simulink model "Hand"  (R2023b)
settings: Solver=ode45  StartTime=0.0  StopTime=100  RelTol=1e-3  EnableMultiTasking=on
model workspace (MAT data in the model file):
  InitialAngle = 0
libraries: simulink x22, vrlib x16, sharedtransform x15
(part 2 of 2)

== system Hand/Subsystem3/Angle To Orientation1 ==
  Y : Inport
  X : Inport  Port=2
  Z : Inport  Port=3
  Multiplier3 : Constant  Value=-1
  Product : Product
  Rotation Angles : Concatenate  NumInputs=3  Mode=Multidimensional array
  Rotation Angles to Direction Cosine Matrix : sharedtransform/Rotation Angles to Direction Cosine Matrix  rotationOrder=XYZ  aMode=aMode
  Rotation Matrix to VR Rotation : vrlib/Utilities/Rotation Matrix to VR Rotation  maxzero=1e-12
  Out1 : Outport
  wires:
  Product/1 -> Rotation Angles to Direction Cosine Matrix/1
  Multiplier3/1 -> Product/1
  Y/1 -> Rotation Angles/2
  Rotation Angles to Direction Cosine Matrix/1 -> Rotation Matrix to VR Rotation/1
  Rotation Matrix to VR Rotation/1 -> Out1/1
  Rotation Angles/1 -> Product/2
  X/1 -> Rotation Angles/1
  Z/1 -> Rotation Angles/3

== system Hand/Subsystem3/Angle To Orientation2 ==
  Y : Inport
  X : Inport  Port=2
  Z : Inport  Port=3
  Multiplier3 : Constant  Value=-1
  Product : Product
  Rotation Angles : Concatenate  NumInputs=3  Mode=Multidimensional array
  Rotation Angles to Direction Cosine Matrix : sharedtransform/Rotation Angles to Direction Cosine Matrix  rotationOrder=XYZ  aMode=aMode
  Rotation Matrix to VR Rotation : vrlib/Utilities/Rotation Matrix to VR Rotation  maxzero=1e-12
  Out1 : Outport
  wires:
  Product/1 -> Rotation Angles to Direction Cosine Matrix/1
  Multiplier3/1 -> Product/1
  Y/1 -> Rotation Angles/2
  Rotation Angles to Direction Cosine Matrix/1 -> Rotation Matrix to VR Rotation/1
  Rotation Matrix to VR Rotation/1 -> Out1/1
  Rotation Angles/1 -> Product/2
  X/1 -> Rotation Angles/1
  Z/1 -> Rotation Angles/3

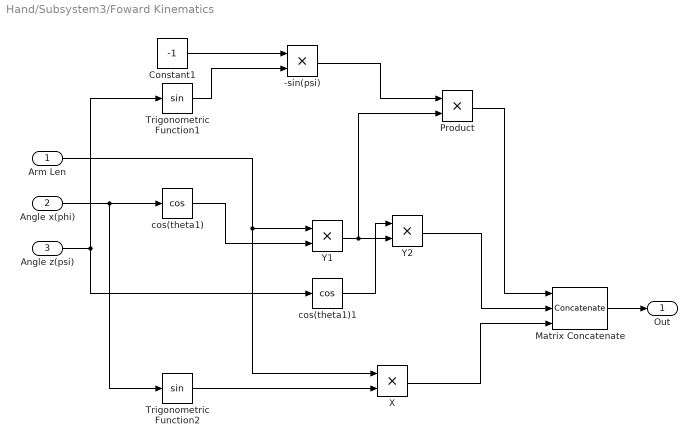
== system Hand/Subsystem3/Foward Kinematics ==
  Arm Len : Inport
  Angle x(phi) : Inport  Port=2
  Angle z(psi) : Inport  Port=3
  -sin(psi) : Product
  Constant1 : Constant  Value=-1
  Matrix Concatenate : Concatenate  NumInputs=3  ConcatenateDimension=2
  Product : Product
  Trigonometric Function1 : Trigonometry  OutputSignalType=real
  Trigonometric Function2 : Trigonometry  OutputSignalType=real
  X : Product
  Y1 : Product
  Y2 : Product
  cos(theta1) : Trigonometry  Operator=cos
  cos(theta1)1 : Trigonometry  Operator=cos
  Out : Outport
  wires:
  Matrix Concatenate/1 -> Out/1
  X/1 -> Matrix Concatenate/3
  Arm Len/1 -> X/1, Y1/1
  Trigonometric Function2/1 -> X/2
  Y1/1 -> Product/2, Y2/2
  cos(theta1)1/1 -> Y2/1
  Y2/1 -> Matrix Concatenate/2
  Product/1 -> Matrix Concatenate/1
  Constant1/1 -> -sin(psi)/1
  Trigonometric Function1/1 -> -sin(psi)/2
  Angle x(phi)/1 -> Trigonometric Function2/1, cos(theta1)/1
  cos(theta1)/1 -> Y1/2
  Angle z(psi)/1 -> Trigonometric Function1/1, cos(theta1)1/1
  -sin(psi)/1 -> Product/1

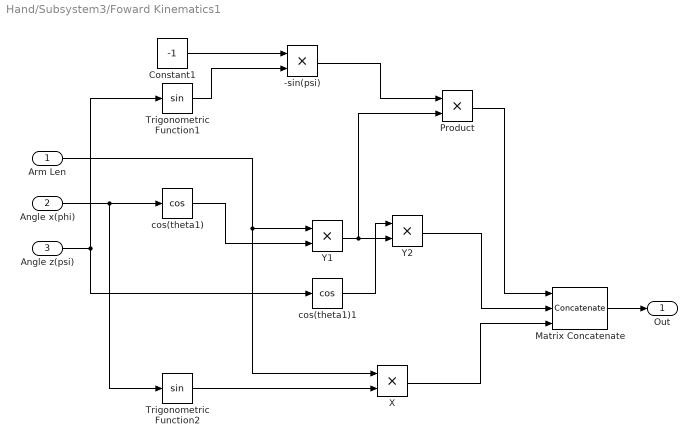
== system Hand/Subsystem3/Foward Kinematics1 ==
  Arm Len : Inport
  Angle x(phi) : Inport  Port=2
  Angle z(psi) : Inport  Port=3
  -sin(psi) : Product
  Constant1 : Constant  Value=-1
  Matrix Concatenate : Concatenate  NumInputs=3  ConcatenateDimension=2
  Product : Product
  Trigonometric Function1 : Trigonometry  OutputSignalType=real
  Trigonometric Function2 : Trigonometry  OutputSignalType=real
  X : Product
  Y1 : Product
  Y2 : Product
  cos(theta1) : Trigonometry  Operator=cos
  cos(theta1)1 : Trigonometry  Operator=cos
  Out : Outport
  wires:
  Matrix Concatenate/1 -> Out/1
  X/1 -> Matrix Concatenate/3
  Arm Len/1 -> X/1, Y1/1
  Trigonometric Function2/1 -> X/2
  Y1/1 -> Product/2, Y2/2
  cos(theta1)1/1 -> Y2/1
  Y2/1 -> Matrix Concatenate/2
  Product/1 -> Matrix Concatenate/1
  Constant1/1 -> -sin(psi)/1
  Trigonometric Function1/1 -> -sin(psi)/2
  Angle x(phi)/1 -> Trigonometric Function2/1, cos(theta1)/1
  cos(theta1)/1 -> Y1/2
  Angle z(psi)/1 -> Trigonometric Function1/1, cos(theta1)1/1
  -sin(psi)/1 -> Product/1

== system Hand/Subsystem4/Angle To Orientation ==
  Y : Inport
  X : Inport  Port=2
  Z : Inport  Port=3
  Multiplier3 : Constant  Value=-1
  Product : Product
  Rotation Angles : Concatenate  NumInputs=3  Mode=Multidimensional array
  Rotation Angles to Direction Cosine Matrix : sharedtransform/Rotation Angles to Direction Cosine Matrix  rotationOrder=XYZ  aMode=aMode
  Rotation Matrix to VR Rotation : vrlib/Utilities/Rotation Matrix to VR Rotation  maxzero=1e-12
  Out1 : Outport
  wires:
  Product/1 -> Rotation Angles to Direction Cosine Matrix/1
  Multiplier3/1 -> Product/1
  Y/1 -> Rotation Angles/2
  Rotation Angles to Direction Cosine Matrix/1 -> Rotation Matrix to VR Rotation/1
  Rotation Matrix to VR Rotation/1 -> Out1/1
  Rotation Angles/1 -> Product/2
  X/1 -> Rotation Angles/1
  Z/1 -> Rotation Angles/3

== system Hand/Subsystem4/Angle To Orientation1 ==
  Y : Inport
  X : Inport  Port=2
  Z : Inport  Port=3
  Multiplier3 : Constant  Value=-1
  Product : Product
  Rotation Angles : Concatenate  NumInputs=3  Mode=Multidimensional array
  Rotation Angles to Direction Cosine Matrix : sharedtransform/Rotation Angles to Direction Cosine Matrix  rotationOrder=XYZ  aMode=aMode
  Rotation Matrix to VR Rotation : vrlib/Utilities/Rotation Matrix to VR Rotation  maxzero=1e-12
  Out1 : Outport
  wires:
  Product/1 -> Rotation Angles to Direction Cosine Matrix/1
  Multiplier3/1 -> Product/1
  Y/1 -> Rotation Angles/2
  Rotation Angles to Direction Cosine Matrix/1 -> Rotation Matrix to VR Rotation/1
  Rotation Matrix to VR Rotation/1 -> Out1/1
  Rotation Angles/1 -> Product/2
  X/1 -> Rotation Angles/1
  Z/1 -> Rotation Angles/3

== system Hand/Subsystem4/Angle To Orientation2 ==
  Y : Inport
  X : Inport  Port=2
  Z : Inport  Port=3
  Multiplier3 : Constant  Value=-1
  Product : Product
  Rotation Angles : Concatenate  NumInputs=3  Mode=Multidimensional array
  Rotation Angles to Direction Cosine Matrix : sharedtransform/Rotation Angles to Direction Cosine Matrix  rotationOrder=XYZ  aMode=aMode
  Rotation Matrix to VR Rotation : vrlib/Utilities/Rotation Matrix to VR Rotation  maxzero=1e-12
  Out1 : Outport
  wires:
  Product/1 -> Rotation Angles to Direction Cosine Matrix/1
  Multiplier3/1 -> Product/1
  Y/1 -> Rotation Angles/2
  Rotation Angles to Direction Cosine Matrix/1 -> Rotation Matrix to VR Rotation/1
  Rotation Matrix to VR Rotation/1 -> Out1/1
  Rotation Angles/1 -> Product/2
  X/1 -> Rotation Angles/1
  Z/1 -> Rotation Angles/3

== system Hand/Subsystem4/Foward Kinematics ==
  Arm Len : Inport
  Angle x(phi) : Inport  Port=2
  Angle z(psi) : Inport  Port=3
  -sin(psi) : Product
  Constant1 : Constant  Value=-1
  Matrix Concatenate : Concatenate  NumInputs=3  ConcatenateDimension=2
  Product : Product
  Trigonometric Function1 : Trigonometry  OutputSignalType=real
  Trigonometric Function2 : Trigonometry  OutputSignalType=real
  X : Product
  Y1 : Product
  Y2 : Product
  cos(theta1) : Trigonometry  Operator=cos
  cos(theta1)1 : Trigonometry  Operator=cos
  Out : Outport
  wires:
  Matrix Concatenate/1 -> Out/1
  X/1 -> Matrix Concatenate/3
  Arm Len/1 -> X/1, Y1/1
  Trigonometric Function2/1 -> X/2
  Y1/1 -> Product/2, Y2/2
  cos(theta1)1/1 -> Y2/1
  Y2/1 -> Matrix Concatenate/2
  Product/1 -> Matrix Concatenate/1
  Constant1/1 -> -sin(psi)/1
  Trigonometric Function1/1 -> -sin(psi)/2
  Angle x(phi)/1 -> Trigonometric Function2/1, cos(theta1)/1
  cos(theta1)/1 -> Y1/2
  Angle z(psi)/1 -> Trigonometric Function1/1, cos(theta1)1/1
  -sin(psi)/1 -> Product/1

== system Hand/Subsystem4/Foward Kinematics1 ==
  Arm Len : Inport
  Angle x(phi) : Inport  Port=2
  Angle z(psi) : Inport  Port=3
  -sin(psi) : Product
  Constant1 : Constant  Value=-1
  Matrix Concatenate : Concatenate  NumInputs=3  ConcatenateDimension=2
  Product : Product
  Trigonometric Function1 : Trigonometry  OutputSignalType=real
  Trigonometric Function2 : Trigonometry  OutputSignalType=real
  X : Product
  Y1 : Product
  Y2 : Product
  cos(theta1) : Trigonometry  Operator=cos
  cos(theta1)1 : Trigonometry  Operator=cos
  Out : Outport
  wires:
  Matrix Concatenate/1 -> Out/1
  X/1 -> Matrix Concatenate/3
  Arm Len/1 -> X/1, Y1/1
  Trigonometric Function2/1 -> X/2
  Y1/1 -> Product/2, Y2/2
  cos(theta1)1/1 -> Y2/1
  Y2/1 -> Matrix Concatenate/2
  Product/1 -> Matrix Concatenate/1
  Constant1/1 -> -sin(psi)/1
  Trigonometric Function1/1 -> -sin(psi)/2
  Angle x(phi)/1 -> Trigonometric Function2/1, cos(theta1)/1
  cos(theta1)/1 -> Y1/2
  Angle z(psi)/1 -> Trigonometric Function1/1, cos(theta1)1/1
  -sin(psi)/1 -> Product/1

== system Hand/Subsystem5/Angle To Orientation ==
  Y : Inport
  X : Inport  Port=2
  Z : Inport  Port=3
  Multiplier3 : Constant  Value=-1
  Product : Product
  Rotation Angles : Concatenate  NumInputs=3  Mode=Multidimensional array
  Rotation Angles to Direction Cosine Matrix : sharedtransform/Rotation Angles to Direction Cosine Matrix  rotationOrder=XYZ  aMode=aMode
  Rotation Matrix to VR Rotation : vrlib/Utilities/Rotation Matrix to VR Rotation  maxzero=1e-12
  Out1 : Outport
  wires:
  Product/1 -> Rotation Angles to Direction Cosine Matrix/1
  Multiplier3/1 -> Product/1
  Y/1 -> Rotation Angles/2
  Rotation Angles to Direction Cosine Matrix/1 -> Rotation Matrix to VR Rotation/1
  Rotation Matrix to VR Rotation/1 -> Out1/1
  Rotation Angles/1 -> Product/2
  X/1 -> Rotation Angles/1
  Z/1 -> Rotation Angles/3

== system Hand/Subsystem5/Angle To Orientation1 ==
  Y : Inport
  X : Inport  Port=2
  Z : Inport  Port=3
  Multiplier3 : Constant  Value=-1
  Product : Product
  Rotation Angles : Concatenate  NumInputs=3  Mode=Multidimensional array
  Rotation Angles to Direction Cosine Matrix : sharedtransform/Rotation Angles to Direction Cosine Matrix  rotationOrder=XYZ  aMode=aMode
  Rotation Matrix to VR Rotation : vrlib/Utilities/Rotation Matrix to VR Rotation  maxzero=1e-12
  Out1 : Outport
  wires:
  Product/1 -> Rotation Angles to Direction Cosine Matrix/1
  Multiplier3/1 -> Product/1
  Y/1 -> Rotation Angles/2
  Rotation Angles to Direction Cosine Matrix/1 -> Rotation Matrix to VR Rotation/1
  Rotation Matrix to VR Rotation/1 -> Out1/1
  Rotation Angles/1 -> Product/2
  X/1 -> Rotation Angles/1
  Z/1 -> Rotation Angles/3

== system Hand/Subsystem5/Angle To Orientation2 ==
  Y : Inport
  X : Inport  Port=2
  Z : Inport  Port=3
  Multiplier3 : Constant  Value=-1
  Product : Product
  Rotation Angles : Concatenate  NumInputs=3  Mode=Multidimensional array
  Rotation Angles to Direction Cosine Matrix : sharedtransform/Rotation Angles to Direction Cosine Matrix  rotationOrder=XYZ  aMode=aMode
  Rotation Matrix to VR Rotation : vrlib/Utilities/Rotation Matrix to VR Rotation  maxzero=1e-12
  Out1 : Outport
  wires:
  Product/1 -> Rotation Angles to Direction Cosine Matrix/1
  Multiplier3/1 -> Product/1
  Y/1 -> Rotation Angles/2
  Rotation Angles to Direction Cosine Matrix/1 -> Rotation Matrix to VR Rotation/1
  Rotation Matrix to VR Rotation/1 -> Out1/1
  Rotation Angles/1 -> Product/2
  X/1 -> Rotation Angles/1
  Z/1 -> Rotation Angles/3

== system Hand/Subsystem5/Foward Kinematics ==
  Arm Len : Inport
  Angle x(phi) : Inport  Port=2
  Angle z(psi) : Inport  Port=3
  -sin(psi) : Product
  Constant1 : Constant  Value=-1
  Matrix Concatenate : Concatenate  NumInputs=3  ConcatenateDimension=2
  Product : Product
  Trigonometric Function1 : Trigonometry  OutputSignalType=real
  Trigonometric Function2 : Trigonometry  OutputSignalType=real
  X : Product
  Y1 : Product
  Y2 : Product
  cos(theta1) : Trigonometry  Operator=cos
  cos(theta1)1 : Trigonometry  Operator=cos
  Out : Outport
  wires:
  Matrix Concatenate/1 -> Out/1
  X/1 -> Matrix Concatenate/3
  Arm Len/1 -> X/1, Y1/1
  Trigonometric Function2/1 -> X/2
  Y1/1 -> Product/2, Y2/2
  cos(theta1)1/1 -> Y2/1
  Y2/1 -> Matrix Concatenate/2
  Product/1 -> Matrix Concatenate/1
  Constant1/1 -> -sin(psi)/1
  Trigonometric Function1/1 -> -sin(psi)/2
  Angle x(phi)/1 -> Trigonometric Function2/1, cos(theta1)/1
  cos(theta1)/1 -> Y1/2
  Angle z(psi)/1 -> Trigonometric Function1/1, cos(theta1)1/1
  -sin(psi)/1 -> Product/1

== system Hand/Subsystem5/Foward Kinematics1 ==
  Arm Len : Inport
  Angle x(phi) : Inport  Port=2
  Angle z(psi) : Inport  Port=3
  -sin(psi) : Product
  Constant1 : Constant  Value=-1
  Matrix Concatenate : Concatenate  NumInputs=3  ConcatenateDimension=2
  Product : Product
  Trigonometric Function1 : Trigonometry  OutputSignalType=real
  Trigonometric Function2 : Trigonometry  OutputSignalType=real
  X : Product
  Y1 : Product
  Y2 : Product
  cos(theta1) : Trigonometry  Operator=cos
  cos(theta1)1 : Trigonometry  Operator=cos
  Out : Outport
  wires:
  Matrix Concatenate/1 -> Out/1
  X/1 -> Matrix Concatenate/3
  Arm Len/1 -> X/1, Y1/1
  Trigonometric Function2/1 -> X/2
  Y1/1 -> Product/2, Y2/2
  cos(theta1)1/1 -> Y2/1
  Y2/1 -> Matrix Concatenate/2
  Product/1 -> Matrix Concatenate/1
  Constant1/1 -> -sin(psi)/1
  Trigonometric Function1/1 -> -sin(psi)/2
  Angle x(phi)/1 -> Trigonometric Function2/1, cos(theta1)/1
  cos(theta1)/1 -> Y1/2
  Angle z(psi)/1 -> Trigonometric Function1/1, cos(theta1)1/1
  -sin(psi)/1 -> Product/1
